simulink model "overhead_crane"  (R2022a)
settings: Solver=ode45  StartTime=0.0  StopTime=50  FixedStep=0.001  MaxStep=0.001  MinStep=0.0001  RelTol=1e-3  AbsTol=0.0001  EnableMultiTasking=on
undefined symbols (not defined in the file): g, k, l, ml, mt, sigbuilder_block
settings Model: Creator=Сергей  LastModifiedBy=clever0ne
settings SolverCC: InitialStep=0.0001  ZeroCrossAlgorithm=Adaptive  AlgebraicLoopSolver=TrustRegion
settings DataIOCC: SaveFormat=Array  ReturnWorkspaceOutputs=off
settings OptimizationCC: LifeSpan=inf
settings DebuggingCC: IgnoredZcDiagnostic=none  UnconnectedInputMsg=warning  UnconnectedOutputMsg=warning  UnconnectedLineMsg=warning  AllowSymbolicDim=off  SFUnexpectedBacktrackingDiag=warning  SFNoUnconditionalDefaultTransitionDiag=warning  SFExecutionAtInitializationDiag=none  SFMachineParentedDataDiag=warning  ArithmeticOperatorsInVariantConditions=warning
settings ModelReferenceCC: PropagateSignalLabelsOutOfModel=off
settings SFSimCC: SimUseLocalCustomCode=off  CustomCodeUndefinedFunction=UseInterfaceOnly
settings RTWCC: RTWUseLocalCustomCode=off
settings CodeAppCC: StateflowObjectComments=on
settings GRTTargetCC: TargetLangStandard=C89/C90 (ANSI)
settings ConfigComp: CovMetricSettings=dw  CovSaveCumulativeToWorkspaceVar=on  CovSaveSingleToWorkspaceVar=on  CovExternalEMLEnable=off

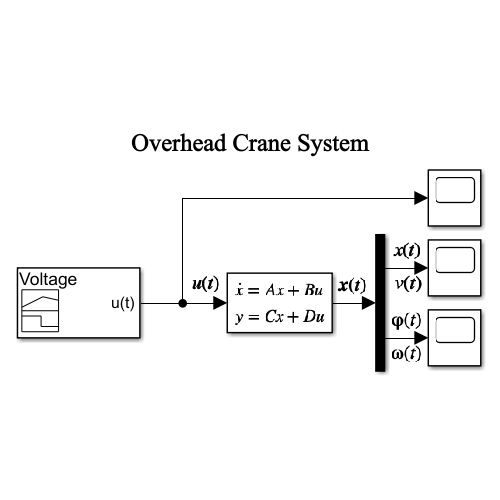
[thumbnail: Simulink's stored preview of the top-level diagram]
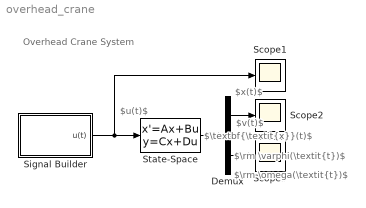
== system overhead_crane ==
  note: $\textbf{\textit{x}}(t)$
  note: Overhead Crane System
  note: $u(t)$
  note: $x(t)$
  note: $\rm \varphi(\textit{t})$
  note: $v(t)$
  note: $\rm \omega(\textit{t})$
  Demux : Demux  Outputs=2
  Scope1 : Scope
  Scope2 : Scope
  Scope3 : Scope
  Signal Builder : Subsystem  Tag=STV Subsys  LoadFcn=sigbuilder_block('load');  StartFcn=sigbuilder_block('start');  StopFcn=sigbuilder_block('stop');  ClipboardFcn=sigbuilder_block('clipboard');  mask(Sigbuilder block){tuvar=[0:10]}
      mask help: Simulink:masks:SigbuilderBlock_MD
      mask init:
      | if ~strcmp(get_param(bdroot(gcbh),'SimulationStatus'),'stopped') tuvar = sigbuilder_block('maskInit'); end
      settings: CopyFcn=sigbuilder_block('copy');  DeleteFcn=sigbuilder_block('delete');  ModelCloseFcn=sigbuilder_block('modelClose');  PreSaveFcn=sigbuilder_block('preSave');  PauseFcn=sigbuilder_block('pause');  ContinueFcn=sigbuilder_block('continue');  NameChangeFcn=sigbuilder_block('namechange');  OpenFcn=sigbuilder_block('open',[207 172.5 550.5 399.75 ]);  CloseFcn=sigbuilder_block('close');
      mask Display: plot(0, 0, 100, 100,[2, 2, 32, 32, 2], [68, 8, 8, 68, 68],[32, 2], [38, 38], [32, 19, 2],[53, 60, 44], [32, 17, 17, 2],[16, 16, 31, 31]);txt = getActiveGroup(gcbh);text(2, 100, txt,'verticalAlignment', 'top');
  State-Space : StateSpace  A=[0, 1, 0, 0; 0, 0, ml*g/mt, 0; 0, 0, 0, 1; 0, 0, -(mt+ml)*g/(mt*l), 0]  B=[0; k/mt; 0; -k/(mt*l)]  C=eye(4)  D=zeros(4, 1)  InitialCondition=0
  wires:
  State-Space/1 -> Demux/1
  Signal Builder/1(u(t)) -> Scope1/1, State-Space/1
  Demux/1 -> Scope2/1
  Demux/2 -> Scope3/1

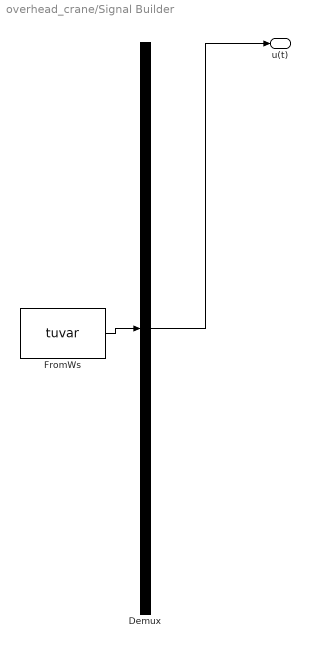
== system overhead_crane/Signal Builder ==
  Demux : Demux  Tag=STV Demux  Outputs=1
      settings: DisplayOption=none
  FromWs : FromWorkspace  Tag=STV FromWs  VariableName=tuvar
      SigBuilderData=|
      | common.afterFinalStr = 'Extrapolate'
      | common.sampleTime = 0
      | dataSet.timeRange = [0 100]
      | dataSet.name = 'Voltage'
      | sbobj.Groups.Name = 'Voltage'
      | sbobj.Groups.Signals.Name = 'u(t)'
      | sbobj.Groups.Signals.XData = [0 1 1 10 10 19 19 100]
      | sbobj.Groups.Signals.YData = [0 0 40 40 -40 -40 0 0]
      | sbobj.Groups.TimeRange = [0 100]
  u(t) : Outport  Tag=STV Outport
  wires:
  Demux/1 -> u(t)/1
  FromWs/1 -> Demux/1
